simulink model "Tra_Los"  (R2016b)
settings: configuration reference "CodeGenConfigSet" (kept outside this file)
values from neighbouring files (symbols this model uses):
  Tra_trqLos_C = Calibration.Parameter    [init_Tra_Los.m]
settings Model: Creator=Colin  LastModifiedBy=Colin
settings ConfigSetRef: SourceLocation=Base Workspace

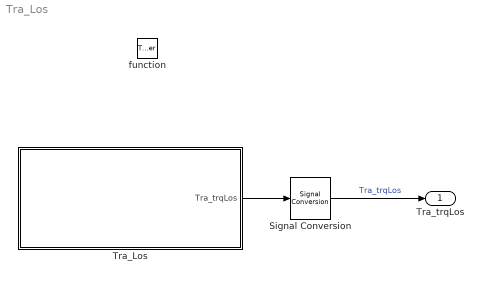
== system Tra_Los ==
  function : TriggerPort  TriggerType=function-call  VariantControl=Variant  PortDimensions=1
  Signal Conversion : SignalConversion  OverrideOpt=off
  Tra_Los : Subsystem
  Tra_trqLos : Outport  Tag=Nm  Description=Gearbox torque loss  OutMin=-3000  OutMax=3000  OutDataTypeStr=Trq_Nm
  wires:
  Tra_Los/1(Tra_trqLos) -> Signal Conversion/1
  Signal Conversion/1 -> Tra_trqLos/1  "Tra_trqLos"

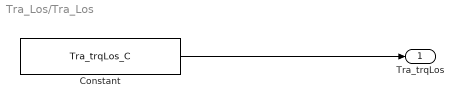
== system Tra_Los/Tra_Los ==
  Constant : Constant  Value=Tra_trqLos_C
  Tra_trqLos : Outport
  wires:
  Constant/1 -> Tra_trqLos/1
